simulink model "sim_parc_fin"  (R2015a)
settings: Solver=ode45  StartTime=0.0  StopTime=600  RelTol=1e-3
values from neighbouring files (symbols this model uses):
  cte = Kp+(Ki/s)+(Kd*s)    [parc final.m]
  G = 0.000002/(s^2+0.01*s+0.0002)    [parc final.m]
libraries: cstblocks x2
settings Model: Creator=Jose Roldan  LastModifiedBy=Jose Roldan

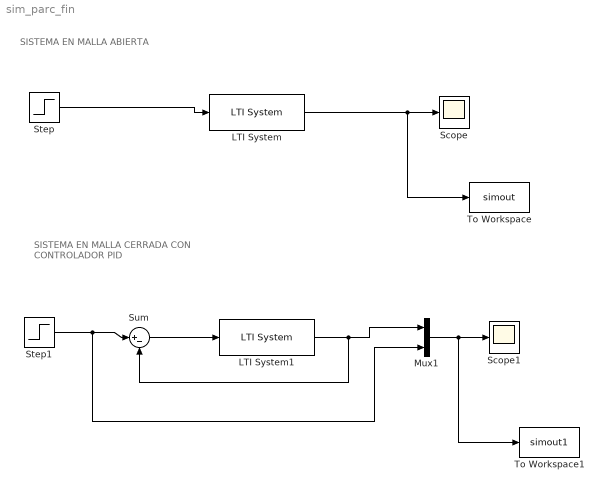
== system sim_parc_fin ==
  note: SISTEMA EN MALLA CERRADA CON
      | CONTROLADOR PID
  note: SISTEMA EN MALLA ABIERTA
  LTI System : cstblocks/LTI System  sys=G  IC=[]
  LTI System1 : cstblocks/LTI System  sys=G*cte  IC=[]
  Mux1 : Mux  Inputs=2
  Scope : Scope
  Scope1 : Scope
  Step : Step  SampleTime=0
  Step1 : Step  SampleTime=0
  Sum : Sum  Inputs=|+-
  To Workspace : ToWorkspace  VariableName=simout  SaveFormat=Timeseries  SampleTime=-1
  To Workspace1 : ToWorkspace  VariableName=simout1  SaveFormat=Timeseries  SampleTime=-1
  wires:
  Step/1 -> LTI System/1
  Sum/1 -> LTI System1/1
  Step1/1 -> Mux1/2, Sum/1
  LTI System1/1 -> Sum/2, Mux1/1
  LTI System/1 -> To Workspace/1, Scope/1
  Mux1/1 -> To Workspace1/1, Scope1/1
